simulink model "ClosedLoop_Stanlay_Controller"  (R2020b)
settings: Solver=VariableStepAuto  StartTime=0.0  StopTime=10  RelTol=1e-3
libraries: simulink x1
settings Model: Creator=99003759  LastModifiedBy=99003759

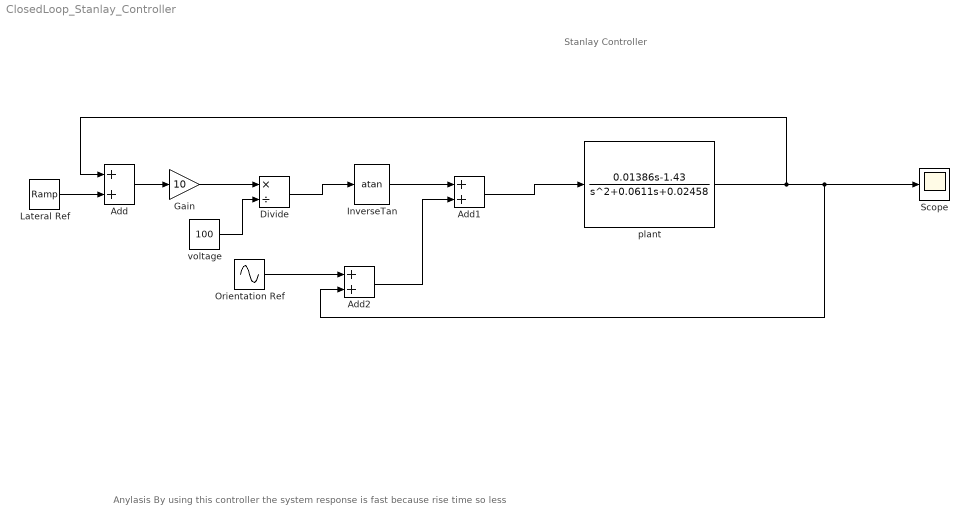
== system ClosedLoop_Stanlay_Controller ==
  note: Anylasis
      | By using this controller the system response is fast because rise time so less
  note: Stanlay Controller
  Add : Sum
  Add1 : Sum
  Add2 : Sum
  Divide : Product  Inputs=*/
  Gain : Gain  Gain=10
  InverseTan : Trigonometry  Operator=atan
  Lateral Ref : simulink/Sources/Ramp  slope=1  start=0  InitialOutput=0
  Orientation Ref : Sin  SampleTime=0
  Scope : Scope
  plant : TransferFcn  Numerator=[0.01386 -1.43]  Denominator=[1 0.0611 0.02458]
  voltage : Constant  Value=100
  wires:
  Add/1 -> Gain/1
  Gain/1 -> Divide/1
  voltage/1 -> Divide/2
  plant/1 -> Add/1, Add2/2, Scope/1
  Divide/1 -> InverseTan/1
  InverseTan/1 -> Add1/1
  Add1/1 -> plant/1
  Add2/1 -> Add1/2
  Orientation Ref/1 -> Add2/1
  Lateral Ref/1 -> Add/2
